simulink model "DrivingScenario"  (R2025b)
settings: Solver=ode1be  StartTime=0  StopTime=200  FixedStep=.01  RelTol=1e-3
model workspace (MAT data in the model file):
  Kd_tbl = '[0.50 0.48 0.45 0.40 0.35 0.32]'
  Kp_tbl = '[8.00 7.50 6.80 5.80 5.00 4.50]'
  Kpsi_tbl = '[1.20 1.25 1.35 1.55 1.75 1.90]'
  Ku = '0.002'
  Ky_tbl = '[0.25 0.22 0.18 0.12 0.09 0.07]'
  L = '2.8'
  Tp = '0.30'
  delta_max = '0.5'
  delta_rate = '0.4'
  tau_d = '0.05'
  torque_max = '8.0'
  v_bp = '[0 5 10 20 30 40]'
undefined symbols (not defined in the file or in its folder): driving, Ki, Kp, Qy, Qyaw, Rang, Sang
libraries: drivingscenarioandsensors x3, simulink x2, simulink_extras x2
settings Model: Creator=Jacob  LastModifiedBy=Sam Ball
settings SFSimCC: SimTargetLang=C++  SimGPUStackLimitPerThread=2048.0  SimDLTargetLibrary=mkl-dnn
settings RTWCC: GPUComputeCapability=3.5

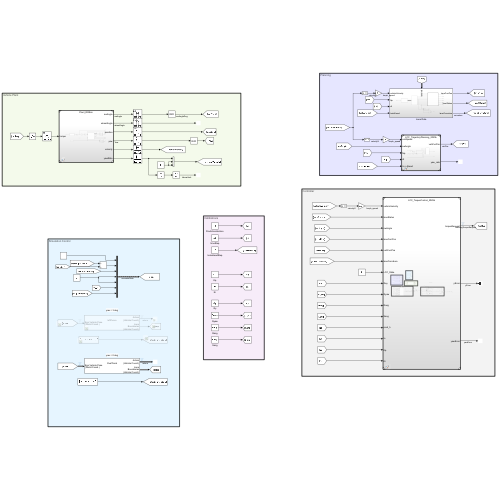
[thumbnail: Simulink's stored preview of the top-level diagram]
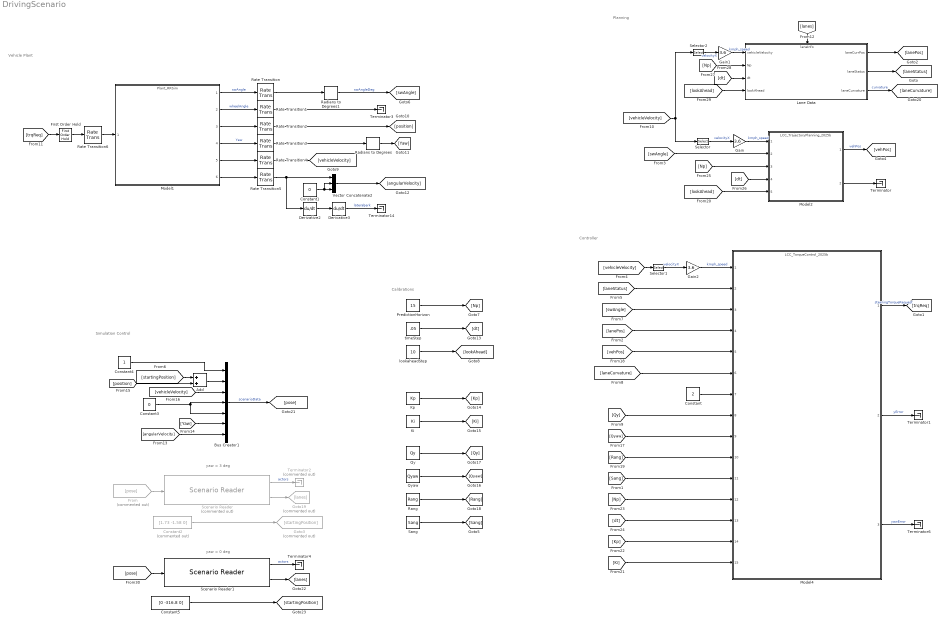
== system DrivingScenario ==
  note: yaw = 0 deg
  note: yaw = 3 deg
  note: Calibrations
  note: Controller
  note: Vehicle Plant
  note: Simulation Control
  note: Planning
  Add : Sum
  Bus Creator1 : BusCreator  Inputs=7  OutDataTypeStr=Bus: BusActorPose  NonVirtualBus=on
      settings: InheritFromInputs=off
  Constant : Constant  Value=2
  Constant1 : Constant  Value=0
  Constant2 : Constant  Commented=on  Value=[1.73 -1.58 0]
  Constant3 : Constant  Value=0
  Constant4 : Constant
  Constant5 : Constant  Value=[0 -316.8 0]
  Derivative2 : Derivative
  Derivative3 : Derivative
  First Order Hold : FirstOrderHold  ErrorTolerance=inf  AllowContinuousInput=on
  From : From  Commented=on  GotoTag=pose
  Gain : Gain  Gain=3.6
  Gain1 : Gain  Gain=3.6
  Gain2 : Gain  Gain=3.6
  Goto19 : Goto  Commented=on  GotoTag=lanes
  Goto3 : Goto  Commented=on  GotoTag=startingPosition
  Ki : Constant  Value=Ki
  Kp : Constant  Value=Kp
  Lane Data : Subsystem
      settings: PortSchema="{\"entries\":[{\"content\":{\"sides\":[{\"content\":{\"connectorIds\":[\"In1\",\"In2\",\"In3\",\"In4\"]},\"type\":\"ConnectorPlacement.EquallySpacedRectSide\",\"uuid\":\"d1d34f75-a798-440a-8d88-70b2a208a78a\"},{\"content\":{\"connectorIds\":[\"Out1\",\"Out2\",\"Out3\"],\"side\":\"RIGHT\"},\"type\":\"ConnectorPlacement.EquallySpacedRectSide\",\"uuid\":\"8445b672-7898-46e0-b896-b3fee4c88930\"},{\"content\":{\"connectorIds\":[\"In5\"],\"side\":\"TOP\"},\"type\":\"ConnectorPlacement.EquallySpacedRectSide\",\"uuid\":\"d2c2deca-5a03-4530-8a19-6a57e3a0b4c3\"}]},\"type\":\"ConnectorPlacement.EquallySpacedConnector\",\"uuid\":\"c994716f-e4a7-413c-899c-7e7da4b03800\"}],\"packageUris\":[\"http://schema.mathworks.com/mf0/Connector/R2020b\"],\"version\":\"1.0\"}"
  Model1 : ModelReference  ModelNameDialog=Plant_RRSim.slx  SimulationMode=Normal  ModelReferenceVersion=5.78
  Model2 : ModelReference  ModelNameDialog=LCC_TrajectoryPlanning_2025b.slx  SimulationMode=Normal  ModelReferenceVersion=5.4
  Model4 : ModelReference  ModelNameDialog=LCC_TorqueControl_2025b.slx  SimulationMode=Normal  ModelReferenceVersion=5.31
  PredictionHorizon : Constant  Value=15
  Qy : Constant  Value=Qy
  Qyaw : Constant  Value=Qyaw
  Radians to Degrees : simulink_extras/Transformations/Radians to Degrees
  Radians to Degrees1 : simulink_extras/Transformations/Radians to Degrees
  Rang : Constant  Value=Rang
  Rate Transition{,1..5} (6 alike) : RateTransition  OutPortSampleTime=simStepSize
  Rate Transition6 : RateTransition  OutPortSampleTime=.01
  Sang : Constant  Value=Sang
  Scenario Reader : drivingscenarioandsensors/Scenario Reader  Commented=on  ScenarioSource=From file  ScenarioFileName=leftCurve.mat  ScenarioVariableName=scenario  OutputCoordinateSystem=Vehicle coordinates  EgoVehicleSource=Input port  EgoVehicleActorID=1  OrientVehiclesOnRoad=off  OutputEgoVehiclePose=off  OutputEgoVehicleState=off  SampleTime=0.05  LaneBoundaryOutput=Ego vehicle lane boundaries  LaneBoundaryDistance=0:0.5:9.5  LaneBoundaryLocation=Center of lane markings  BusNameSource=Auto  BusName=BusActors  BusNumActorsSource=Scenario  BusNumActors=100  BusName2Source=Auto  BusName2=BusLaneBoundaries  BusNumLaneBoundariesSource=Scenario  BusNumLaneBoundaries=10  BusName3Source=Auto  BusName3=BusEgoActor  BusName4Source=Auto  BusName4=BusEgoState  ShowCoordinateLabels=on  SimulateUsing=Interpreted execution
  Scenario Reader1 : drivingscenarioandsensors/Scenario Reader  ScenarioSource=From file  ScenarioFileName=OvalTrack.mat  ScenarioVariableName=scenario  OutputCoordinateSystem=Vehicle coordinates  EgoVehicleSource=Input port  EgoVehicleActorID=1  OrientVehiclesOnRoad=off  OutputEgoVehiclePose=off  OutputEgoVehicleState=off  SampleTime=0.05  LaneBoundaryOutput=Ego vehicle lane boundaries  LaneBoundaryDistance=0:0.5:9.5  LaneBoundaryLocation=Center of lane markings  BusNameSource=Auto  BusName=BusActors  BusNumActorsSource=Scenario  BusNumActors=100  BusName2Source=Auto  BusName2=BusLaneBoundaries  BusNumLaneBoundariesSource=Scenario  BusNumLaneBoundaries=10  BusName3Source=Auto  BusName3=BusEgoActor  BusName4Source=Auto  BusName4=BusEgoState  ShowCoordinateLabels=on  SimulateUsing=Interpreted execution
  Selector : Selector  InputPortWidth=3  IndexOptions=Index vector (dialog)  Indices=1  OutputSizes=1
  Selector1 : Selector  InputPortWidth=3  IndexOptions=Index vector (dialog)  Indices=1  OutputSizes=1
  Selector2 : Selector  InputPortWidth=3  IndexOptions=Index vector (dialog)  Indices=1  OutputSizes=1
  Terminator{,1,3..4,6,14} (6 alike) : Terminator
  Terminator2 : Terminator  Commented=on
  Vector Concatenate2 : Concatenate  NumInputs=3  Mode=Multidimensional array  ConcatenateDimension=2
  lookaheadStep : Constant  Value=10
  timeStep : Constant  Value=.05
  wires:
  Radians to Degrees1/1 -> [swAngle]  "swAngleDeg"
  [Yaw] -> Bus Creator1/6
  Model1/4 -> Rate Transition3/1  "Yaw"
  Derivative2/1 -> Derivative3/1
  Model1/1 -> Rate Transition/1  "swAngle"
  Radians to Degrees/1 -> [Yaw]
  Model2/1 -> [vehPos]  "vehPos"
  [vehicleVelocity] -> Selector/1, Selector2/1
  Vector Concatenate2/1 -> [angularVelocity]
  Model1/2 -> Rate Transition1/1  "wheelAngle"
  Constant1/1 -> Vector Concatenate2/2, Vector Concatenate2/3
  [vehicleVelocity] -> Bus Creator1/3
  Derivative3/1 -> Terminator14/1  "lateralJerk"
  [angularVelocity] -> Bus Creator1/7
  [trqReq] -> First Order Hold/1
  Lane Data/2(laneStatus) -> [laneStatus]
  Selector/1 -> Gain/1  "velocityX"
  Gain/1 -> Model2/1  "kmph_speed"
  [swAngle] -> Model2/2
  Lane Data/1(laneCurrPos) -> [lanePos]
  [vehicleVelocity] -> Selector1/1
  Selector1/1 -> Gain2/1  "velocityX"
  [Np] -> Model2/3
  [dt] -> Model2/4
  Rang/1 -> [Rang]
  Qyaw/1 -> [Qyaw]
  Qy/1 -> [Qy]
  Ki/1 -> [Ki]
  Kp/1 -> [Kp]
  timeStep/1 -> [dt]
  PredictionHorizon/1 -> [Np]
  [Np] -> Lane Data/2(Np)
  [dt] -> Lane Data/3(dt)
  Model4/1 -> [trqReq]  "steeringTorqueRequest"
  Selector2/1 -> Gain1/1  "velocityX"
  Gain1/1 -> Lane Data/1(vehicleVelocity)  "kmph_speed"
  [position] -> Add/2
  Add/1 -> Bus Creator1/2
  [startingPosition] -> Add/1
  Sang/1 -> [Sang]
  Lane Data/3(laneCurvature) -> [laneCurvature]  "curvature"
  Model2/2 -> Terminator/1
  Model4/2 -> Terminator1/1  "yError"
  Model4/3 -> Terminator6/1  "yawError"
  Gain2/1 -> Model4/1  "kmph_speed"
  [laneStatus] -> Model4/2
  [swAngle] -> Model4/3
  [lanePos] -> Model4/4
  [vehPos] -> Model4/5
  [laneCurvature] -> Model4/6
  Constant/1 -> Model4/7
  [Qy] -> Model4/8
  [Qyaw] -> Model4/9
  [Rang] -> Model4/10
  [Sang] -> Model4/11
  [Np] -> Model4/12
  [dt] -> Model4/13
  [Kp] -> Model4/14
  [Ki] -> Model4/15
  Constant3/1 -> Bus Creator1/5, Bus Creator1/4
  Constant4/1 -> Bus Creator1/1
  Scenario Reader/1 -> Terminator2/1  "actors"
  Scenario Reader/2 -> Goto19/1
  Bus Creator1/1 -> [pose]  "scenarioData"
  From/1 -> Scenario Reader/1
  [lanes] -> Lane Data/5(laneInfo)
  First Order Hold/1 -> Rate Transition6/1
  Model1/3 -> Rate Transition2/1
  Model1/5 -> Rate Transition4/1
  Model1/6 -> Rate Transition5/1
  Rate Transition/1 -> Radians to Degrees1/1
  Rate Transition1/1 -> Terminator3/1
  Rate Transition2/1 -> [position]
  Rate Transition3/1 -> Radians to Degrees/1
  Rate Transition4/1 -> [vehicleVelocity]
  Rate Transition5/1 -> Derivative2/1, Vector Concatenate2/1
  Rate Transition6/1 -> Model1/1
  lookaheadStep/1 -> [lookAhead]
  [lookAhead] -> Model2/5
  [lookAhead] -> Lane Data/4(lookAhead)
  Constant2/1 -> Goto3/1
  Scenario Reader1/1 -> Terminator4/1  "actors"
  Constant5/1 -> [startingPosition]
  [pose] -> Scenario Reader1/1
  Scenario Reader1/2 -> [lanes]

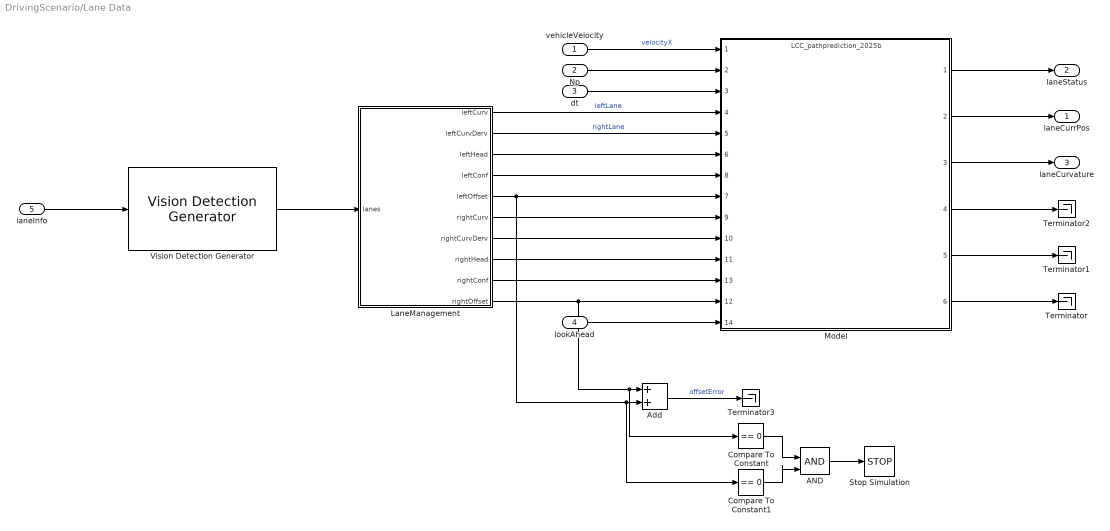
== system DrivingScenario/Lane Data ==
  vehicleVelocity : Inport
  Np : Inport  Port=2
  dt : Inport  Port=3
  lookAhead : Inport  Port=4
  laneInfo : Inport  Port=5
  AND : Logic  IconShape=distinctive  AllPortsSameDT=off  OutDataTypeStr=boolean
  Add : Sum
  Compare To Constant : simulink/Logic and Bit Operations/Compare To Constant  relop===  const=0  OutDataTypeStr=boolean
  Compare To Constant1 : simulink/Logic and Bit Operations/Compare To Constant  relop===  const=0  OutDataTypeStr=boolean
  LaneManagement : MATLAB Function  TreatAsAtomicUnit=on
  Model : ModelReference  ModelNameDialog=LCC_pathprediction_2025b.slx  SimulationMode=Normal  ModelReferenceVersion=5.5
      settings: PortSchema="{\"entries\":[{\"content\":{\"sides\":[{\"content\":{\"connectorIds\":[\"In1\",\"In2\",\"In3\",\"In4\",\"In5\",\"In6\",\"In8\",\"In7\",\"In9\",\"In10\",\"In11\",\"In13\",\"In12\",\"In14\"]},\"type\":\"ConnectorPlacement.EquallySpacedRectSide\",\"uuid\":\"a74d81f4-c7d7-4804-a14b-01728b6478f5\"},{\"content\":{\"connectorIds\":[\"Out1\",\"Out2\",\"Out3\",\"Out4\",\"Out5\",\"Out6\"],\"side\":\"RIGHT\"},\"type\":\"ConnectorPlacement.EquallySpacedRectSide\",\"uuid\":\"21126dcf-3775-4261-ae5e-6e1eba38ba94\"},{\"content\":{\"side\":\"TOP\"},\"type\":\"ConnectorPlacement.EquallySpacedRectSide\",\"uuid\":\"dd74ba6d-3383-4e3a-8460-e981e64bdeb5\"}]},\"type\":\"ConnectorPlacement.EquallySpacedConnector\",\"uuid\":\"d3dbcf7d-fd05-4c31-b3b9-7a7500a66aa5\"}],\"packageUris\":[\"http://schema.mathworks.com/mf0/Connector/R2020b\"],\"version\":\"1.0\"}"
  Stop Simulation : Stop
  Terminator{,1..3} (4 alike) : Terminator
  Vision Detection Generator : drivingscenarioandsensors/Vision Detection Generator  SensorIndex=1  DetectorOutput=Lanes only  UpdateInterval=simStepSize  LaneUpdateInterval=simStepSize  SensorLocation=[ 1, 0 ]  Height=1.9  Yaw=0  Pitch=1  Roll=0  BusNameSource=Auto  BusName=BusObjectDetections  BusName2Source=Auto  BusName2=BusLaneDetections  MaxNumDetectionsSource=Property  MaxNumDetections=10  MaxNumLanesSource=Property  MaxNumLanes=4  DetectionCoordinates=Ego Cartesian  SimulateUsing=Code generation  MaxRange=100  BoundingBoxAccuracy=5  ProcessNoiseIntensity=5  MaxSpeed=100  MaxAllowedOcclusion=0.5  MinObjectImageSize=[ 5, 5 ]  DetectionProbability=0.99  FalsePositivesPerImage=0.01  MinLaneImageSize=[ 20, 3 ]  LaneBoundaryAccuracy=3  HasNoise=off  InitialSeedSource=Not repeatable  InitialSeed=0  UsedSeed=driving.internal.SimulinkUtilities.seedManager(gcb)  ActorProfilesSource=From Scenario Reader block  ActorProfilesParameters=driving.internal.ActorProfilesParameters  ActorProfilesExpression=struct( 'ClassID', 0, 'Length', 4.7, 'Width', 1.8, 'Height', 1.4, 'OriginOffset', [ -1.35, 0, 0 ] )  Intrinsics=driving.internal.cameraIntrinsics
  laneCurrPos : Outport
  laneStatus : Outport  Port=2
  laneCurvature : Outport  Port=3
  wires:
  laneInfo/1 -> Vision Detection Generator/1
  Vision Detection Generator/1 -> LaneManagement/1(lanes)
  Model/1 -> laneStatus/1
  Model/2 -> laneCurrPos/1
  vehicleVelocity/1 -> Model/1  "velocityX"
  Np/1 -> Model/2
  dt/1 -> Model/3
  LaneManagement/1(leftCurv) -> Model/4  "leftLane"
  LaneManagement/2(leftCurvDerv) -> Model/5  "rightLane"
  LaneManagement/3(leftHead) -> Model/6
  LaneManagement/4(leftConf) -> Model/8
  LaneManagement/5(leftOffset) -> Compare To Constant1/1, Add/2, Model/7
  LaneManagement/6(rightCurv) -> Model/9
  LaneManagement/10(rightOffset) -> Compare To Constant/1, Add/1, Model/12
  LaneManagement/9(rightConf) -> Model/13
  LaneManagement/8(rightHead) -> Model/11
  LaneManagement/7(rightCurvDerv) -> Model/10
  Add/1 -> Terminator3/1  "offsetError"
  Model/3 -> laneCurvature/1
  Model/4 -> Terminator2/1
  Model/5 -> Terminator1/1
  Model/6 -> Terminator/1
  lookAhead/1 -> Model/14
  Compare To Constant/1 -> AND/1
  Compare To Constant1/1 -> AND/2
  AND/1 -> Stop Simulation/1

== matlab function DrivingScenario/Lane Data/LaneManagement ==
  data: lanes input; leftCurv output; leftCurvDerv output; leftHead output; leftConf output; leftOffset output; rightCurv output; rightCurvDerv output; rightHead output; rightConf output; rightOffset output
function [leftCurv, leftCurvDerv, leftHead, leftConf, leftOffset, rightCurv, rightCurvDerv, rightHead, rightConf, rightOffset] = LaneManagement(lanes)

leftCurv = 0;
leftCurvDerv = 0;
leftHead = 0;
leftConf = 0;
leftOffset = 0;

rightCurv = 0;
rightCurvDerv = 0;
rightHead = 0;
rightConf = 0;
rightOffset = 0;

for i=1:lanes.NumLaneBoundaries
    
    if (lanes.LaneBoundaries(i).LateralOffset > 0) && (lanes.LaneBoundaries(i).LateralOffset < 2.5)
        leftCurv = double(lanes.LaneBoundaries(i).Curvature);
        leftCurvDerv = double(lanes.LaneBoundaries(i).CurvatureDerivative);
        leftHead = deg2rad(double(lanes.LaneBoundaries(i).HeadingAngle));
        leftOffset = double(lanes.LaneBoundaries(i).LateralOffset);
        leftConf = double(1);

    elseif (lanes.LaneBoundaries(i).LateralOffset < 0) && (lanes.LaneBoundaries(i).LateralOffset > -2.5)
        rightCurv = double(lanes.LaneBoundaries(i).Curvature);
        rightCurvDerv = double(lanes.LaneBoundaries(i).CurvatureDerivative);
        rightHead = deg2rad(double(lanes.LaneBoundaries(i).HeadingAngle));
        rightOffset = double(lanes.LaneBoundaries(i).LateralOffset);
        rightConf = double(1);
    end


    %negative lateral offset if right lane
end
